simulink model "PMSM_Drive_custom_pwm"  (R2019b)
settings: Solver=VariableStepAuto  StartTime=0.0  StopTime=0.5  MaxStep=1e-6  RelTol=1e-3
undefined symbols (not defined in the file): f_sw, U_DC
libraries: controllers x2, coordinate_transformations x2, PE_components x1
settings Model: SimulationMode=accelerator  Creator=kissd  LastModifiedBy=kissd

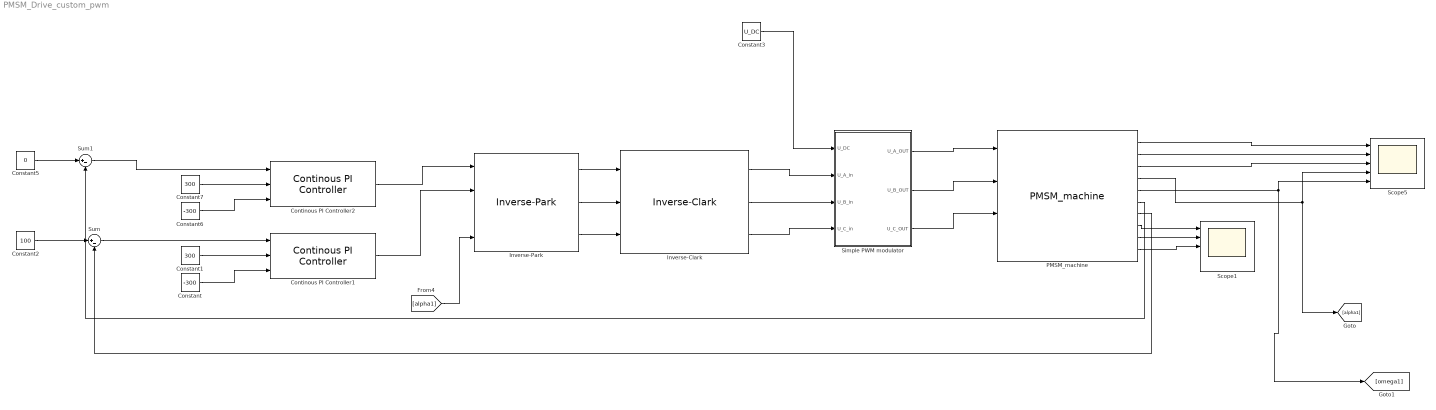
== system PMSM_Drive_custom_pwm ==
  Constant : Constant  Value=-300
  Constant1 : Constant  Value=300
  Constant2 : Constant  Value=100
  Constant3 : Constant  Value=U_DC
  Constant5 : Constant  Value=0
  Constant6 : Constant  Value=-300
  Constant7 : Constant  Value=300
  Continous PI Controller1 : controllers/Continous PI Controller  Ap=Ap  Ti=Ti
  Continous PI Controller2 : controllers/Continous PI Controller  Ap=Ap  Ti=Ti
  Inverse-Clark : coordinate_transformations/Inverse-Clark  SystemSampleTime=-1  Latency=0  AutoFrameSizeCalculation=off
  Inverse-Park : coordinate_transformations/Inverse-Park  SystemSampleTime=-1  Latency=0  AutoFrameSizeCalculation=off
  PMSM_machine : PE_components/PMSM_machine  SystemSampleTime=-1  Latency=0  AutoFrameSizeCalculation=off
      link override Gain: Gain=1/Ld
      link override Gain1: Gain=Rs
      link override Gain2: Gain=Rs
      link override Gain4: Gain=1/Theta
      link override Gain7: Gain=3/2
      link override Integrator2: InitialCondition=0
      link override Sum2: Inputs=++-
  Scope1 : Scope  NumInputPorts=5
  Scope5 : Scope  NumInputPorts=5
  Simple PWM modulator : Subsystem
  Sum : Sum  Inputs=|+-
  Sum1 : Sum  Inputs=|+-
  wires:
  PMSM_machine/2 -> Scope5/2
  PMSM_machine/3 -> Scope5/3
  PMSM_machine/1 -> Scope5/1
  PMSM_machine/4 -> [alpha1], Scope5/4
  PMSM_machine/5 -> [omega1], Scope5/5
  Constant3/1 -> Simple PWM modulator/1(U_DC)
  Inverse-Park/2 -> Inverse-Clark/2
  Inverse-Park/1 -> Inverse-Clark/1
  Inverse-Park/3 -> Inverse-Clark/3
  [alpha1] -> Inverse-Park/4
  Constant2/1 -> Sum/1
  Constant/1 -> Continous PI Controller1/3
  Constant1/1 -> Continous PI Controller1/2
  Sum/1 -> Continous PI Controller1/1
  PMSM_machine/7 -> Sum/2
  Continous PI Controller1/1 -> Inverse-Park/2
  Constant7/1 -> Continous PI Controller2/2
  Constant6/1 -> Continous PI Controller2/3
  Sum1/1 -> Continous PI Controller2/1
  Continous PI Controller2/1 -> Inverse-Park/1
  Constant5/1 -> Sum1/1
  PMSM_machine/6 -> Sum1/2
  Inverse-Clark/3 -> Simple PWM modulator/4(U_C_in)
  Inverse-Clark/2 -> Simple PWM modulator/3(U_B_in)
  Inverse-Clark/1 -> Simple PWM modulator/2(U_A_in)
  Simple PWM modulator/1(U_A_OUT) -> PMSM_machine/1
  Simple PWM modulator/2(U_B_OUT) -> PMSM_machine/2
  Simple PWM modulator/3(U_C_OUT) -> PMSM_machine/3
  PMSM_machine/8 -> Scope1/1
  PMSM_machine/9 -> Scope1/2
  PMSM_machine/10 -> Scope1/3

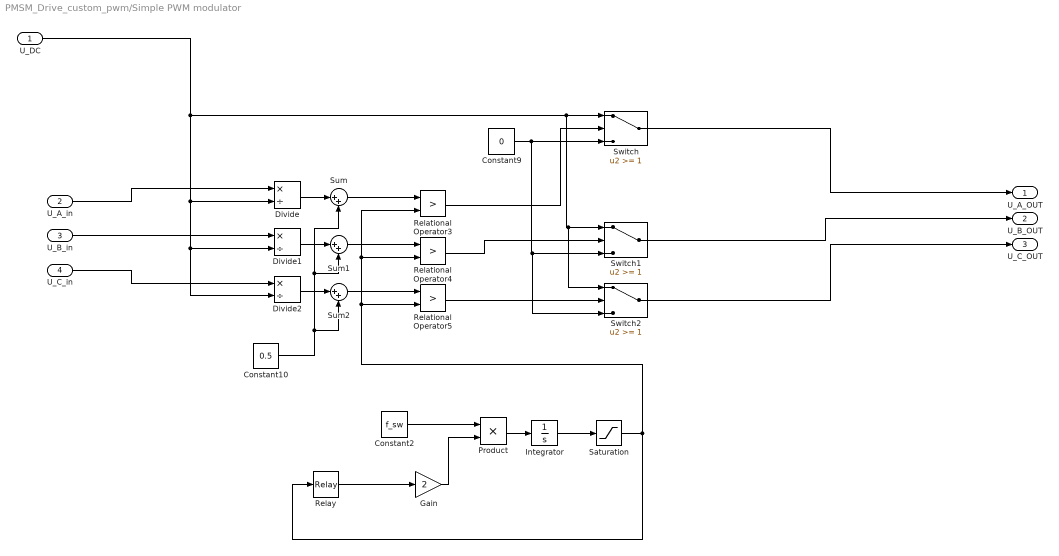
== system PMSM_Drive_custom_pwm/Simple PWM modulator ==
  U_DC : Inport
  U_A_in : Inport  Port=2
  U_B_in : Inport  Port=3
  U_C_in : Inport  Port=4
  Constant10 : Constant  Value=0.5
  Constant2 : Constant  Value=f_sw
  Constant9 : Constant  Value=0
  Divide : Product  Inputs=*/
  Divide1 : Product  Inputs=*/
  Divide2 : Product  Inputs=*/
  Gain : Gain  Gain=2
  Integrator : Integrator
  Product : Product
  Relational Operator3 : RelationalOperator  Operator=>  OutDataTypeStr=boolean  RndMeth=Simplest
  Relational Operator4 : RelationalOperator  Operator=>  OutDataTypeStr=boolean  RndMeth=Simplest
  Relational Operator5 : RelationalOperator  Operator=>  OutDataTypeStr=boolean  RndMeth=Simplest
  Relay : Relay  OnSwitchValue=1  OffSwitchValue=0  OnOutputValue=-1  OffOutputValue=1
  Saturation : Saturate  UpperLimit=1  LowerLimit=0
  Sum : Sum  Inputs=|++
  Sum1 : Sum  Inputs=|++
  Sum2 : Sum  Inputs=|++
  Switch : Switch  Threshold=1
  Switch1 : Switch  Threshold=1
  Switch2 : Switch  Threshold=1
  U_A_OUT : Outport
  U_B_OUT : Outport  Port=2
  U_C_OUT : Outport  Port=3
  wires:
  Constant2/1 -> Product/1
  Sum1/1 -> Relational Operator4/1
  Product/1 -> Integrator/1
  Relational Operator5/1 -> Switch2/2
  U_DC/1 -> Divide2/2, Divide1/2, Divide/2, Switch2/1, Switch1/1, Switch/1
  Integrator/1 -> Saturation/1
  Divide1/1 -> Sum1/1
  Saturation/1 -> Relay/1, Relational Operator3/2, Relational Operator4/2, Relational Operator5/2
  Relay/1 -> Gain/1
  Constant10/1 -> Sum2/2, Sum1/2, Sum/2
  Relational Operator3/1 -> Switch/2
  Switch/1 -> U_A_OUT/1
  U_B_in/1 -> Divide1/1
  Switch2/1 -> U_C_OUT/1
  Constant9/1 -> Switch2/3, Switch1/3, Switch/3
  Relational Operator4/1 -> Switch1/2
  Gain/1 -> Product/2
  Sum/1 -> Relational Operator3/1
  Divide2/1 -> Sum2/1
  Divide/1 -> Sum/1
  Sum2/1 -> Relational Operator5/1
  U_C_in/1 -> Divide2/1
  U_A_in/1 -> Divide/1
  Switch1/1 -> U_B_OUT/1
